simulink library "RoboticsPlayground"  (R2021a)
settings: Solver=FixedStepDiscrete  StartTime=0.0  StopTime=10.0  FixedStep=0.01  RelTol=1e-3
InitFcn:
  | RPInit
undefined symbols (not defined in the file or in its folder): Base, ChassisCOG, Claw2Block1, Claw2Block2, FloorSurface, Frame, PlowSurface, Ref, RobotSurface, Side1, Side2, Wheel2Ground, X, Y, Z
libraries: sm_lib x198, nesl_utility x43, RP_Simulator_Components x23, simulink x2, pid_lib x1
(part 1 of 7)
settings Model: Creator=josea  LastModifiedBy=Sebastian
settings SolverCC: AlgebraicLoopSolver=TrustRegion
settings DataIOCC: ReturnWorkspaceOutputs=off
settings DebuggingCC: SFMachineParentedDataDiag=warning  ArithmeticOperatorsInVariantConditions=warning
settings SFSimCC: SimUseLocalCustomCode=off  CustomCodeUndefinedFunction=UseInterfaceOnly
settings RTWCC: RTWUseLocalCustomCode=off

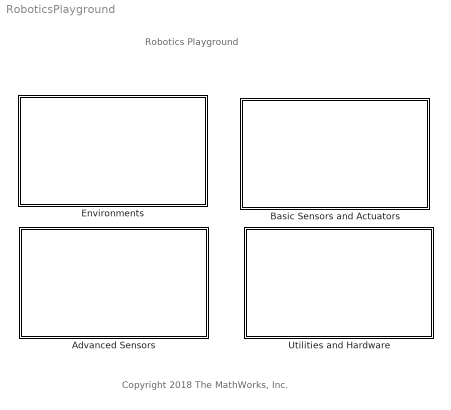
== system RoboticsPlayground ==
  note: Robotics Playground
  note: Copyright 2018 The MathWorks, Inc.
  Advanced Sensors : Subsystem
      mask Display: image('advanced_sensors_lib.PNG')
  Basic Sensors and Actuators : Subsystem
      mask Display: image('sensors_lib.PNG')
  Environments : Subsystem
      mask Display: image('environments_lib.PNG')
  Utilities and Hardware : Subsystem

== system RoboticsPlayground/Advanced Sensors ==
  note: Advanced Sensors
      |
      | Use one of this blocks for each device
  360 Range Sensor : Subsystem  mask(RP 360 Sensor){robotId=1, maxSenRange=2, sensOff=[0 0], sensDegRes=1, sensorTs=0.1}
      mask prompts: robotId "Robot ID"; maxSenRange "Maximum Range (m)"; sensOff "Sensor Position Offset X Y [m]"; sensDegRes "Angular Resolution [deg]"; sensorTs "Sensor sample time [s]"
      mask help:
      | This sensor outputs the ranges measured by a distance sensor at multiple angles of rotation. This sensor can detect walls and obstacles within the simulation environments.
      |
      | The block outputs an array with variable dimensions depending and corresponding to the angular sensor resolution. An angular resolution of 1 degree means the block will output an array of 360 elements each corresponding to the respective ranges at angles from 0 to 359 degrees.
      |
      | NOTE: This block has no visualization in the virtual environment.
      mask init:
      | ID=get_param(gcb,'robotId');
      | 
      | set_param([gcb '/xPose'],'GotoTag',['R' ID 'xPose']);
      | set_param([gcb '/yPose'],'GotoTag',['R' ID 'yPose']);
      | set_param([gcb '/tPose'],'GotoTag',['R' ID 'tPose']);
      mask Help: web('360_sensor.htm')
      mask DialogControl senCont Prompt: Sensor Characteristics
      mask Display:
      | color('white');
      | plot([100,100,100,100]*1,[100,100,100,100]*1);
      | plot([100,100,100,100]*0,[100,100,100,100]*0);
      | image('Lidar.png')
      | color('blue');
      | id=eval(get_param(gcb,'robotId'));
      | text(99, 92, ['Robot ID: ' num2str(id)], 'horizontalAlignment', 'right');
  Object Detector : Subsystem  mask(RP Object Sensor){robotId=1, maxSenRange=2, sensFOV=90, sensOff=[0 0], sensOffDeg=0, sensorTs=0.1}
      mask prompts: robotId "Robot ID"; maxSenRange "Maximum Range (m)"; sensFOV "Sensor Field of View [deg]"; sensOff "Sensor Position Offset X Y [m]"; sensOffDeg "Sensor Orientation Offset [deg]"; sensorTs "Sensor sample time [s]"
      mask help:
      | This block returns information from all the objects that are in the field of vision of the sensor.
      |
      | The output of this block is a variable sized depending on the number of objects that are in sight.
      |
      | This block outputs the [ranges angles labels] of the identified objects. Use the "Pick color" block in the Robotics Playground library to obtain information about a single object.
      |
      | Please refer to the detailed documentation by pressing the "Help" button.
      mask init:
      | ID=get_param(gcb,'robotId');
      | 
      | set_param([gcb '/xPose'],'GotoTag',['R' ID 'xPose']);
      | set_param([gcb '/yPose'],'GotoTag',['R' ID 'yPose']);
      | set_param([gcb '/tPose'],'GotoTag',['R' ID 'tPose']);
      mask Help: web('object_sensor.htm')
      mask DialogControl senCont Prompt: Sensor Characteristics
      mask Display:
      | color('white');
      | plot([100,100,100,100]*1,[100,100,100,100]*1);
      | plot([100,100,100,100]*0,[100,100,100,100]*0);
      | image('ObjectDetector.png','center')
      | color('blue');
      | id=eval(get_param(gcb,'robotId'));
      | text(99, 92, ['Robot ID: ' num2str(id)], 'horizontalAlignment', 'right');
      | color('black')
      | port_label('output', 1', 'Objects');
  Pick Color : Subsystem  mask(RP Pick Color){colorSelection=Red}
      mask prompts: colorSelection "Color"
      mask help: This block receives all the detections from the output of a RP Object Detector and outputs the angle in degrees and distance in meters to the nearest object of the selected color.
      mask init:
      | colorSelection=get_param(gcb,'colorSelection');
      | 
      | if strcmp(colorSelection,'Red')
      |     color=1;
      | elseif strcmp(colorSelection,'Green')
      |     color=2;
      | else
      |     color=3;
      | end
      mask Help: web('pick_color.htm')
      mask TypeOptions colorSelection: Red | Green | Blue
      mask Display:
      | colorSelection=get_param(gcb,'colorSelection');
      | 
      | if strcmp(colorSelection,'Red')
      |     image('RedObjD.png','center')
      | elseif strcmp(colorSelection,'Green')
      |     image('GreenObjD.png','center')
      | else
      |     image('BlueObjD.png','center')
      | end
      | 
      | color('black');
      | port_label('input', 1', 'Objects');
      | port_label('output', 1', 'Angle');
      | port_label('output', 2', 'Distance');

== system RoboticsPlayground/Basic Sensors and Actuators ==
  note: Basic Sensors and Actuators
      |
      | Use one of this blocks for each device
  Compass Sensor : Subsystem  mask(RP Compass Sensor){robotId=1, sensorTs=0.1}
      mask prompts: robotId "Robot ID"; sensorTs "Sensor sample time [s]"
      mask help: This sensor outputs the rotation in degrees as measured from the robot center relative to the world coordinate frame.
      mask init:
      | ID=get_param(gcb,'robotId');
      | 
      | set_param([gcb '/tRate'],'GotoTag',['R' ID 'tAngle']);
      mask Help: web('compass_sensor.htm')
      mask DialogControl senCont Prompt: Sensor Characteristics
      mask Display:
      | color('white');
      | plot([100,100,100,100]*1,[100,100,100,100]*1);
      | plot([100,100,100,100]*0,[100,100,100,100]*0);
      | image('Compass.png','center')
      | color('blue');
      | id=eval(get_param(gcb,'robotId'));
      | text(99, 92, ['Robot ID: ' num2str(id)], 'horizontalAlignment', 'right');
  Contact Switch : Subsystem  mask(RP Contact Switch){robotId=1, trigDist=0.02, sensOff=[0 0], sensOffDeg=0, sensorTs=0.1}
      mask prompts: robotId "Robot ID"; trigDist "Trigger Distance [m]"; sensOff "Sensor Position Offset X Y [m]"; sensOffDeg "Sensor Orientation Offset [deg]"; sensorTs "Sensor sample time [s]"
      mask help:
      | This block outputs 1 if the sensor comes in close proximity to a wall or obstacle. Otherwise it outputs zero. The proximity at which the sensor is triggered can be set through the mask using the "Trigger Distance" field. Default values can also be used.
      |
      | Sensor position and orientation offsets are with respect to the robot center.
      mask init:
      | ID=get_param(gcb,'robotId');
      | 
      | set_param([gcb '/xPose'],'GotoTag',['R' ID 'xPose']);
      | set_param([gcb '/yPose'],'GotoTag',['R' ID 'yPose']);
      | set_param([gcb '/tPose'],'GotoTag',['R' ID 'tPose']);
      mask Help: web('contact_switch.htm')
      mask DialogControl senCont Prompt: Sensor Characteristics
      mask Display:
      | color('white');
      | plot([100,100,100,100]*1,[100,100,100,100]*1);
      | plot([100,100,100,100]*0,[100,100,100,100]*0);
      | image('ContactSwitch.png','center')
      | color('blue');
      | id=eval(get_param(gcb,'robotId'));
      | text(99, 92, ['Robot ID: ' num2str(id)], 'horizontalAlignment', 'right');
  Distance Sensor : Subsystem  mask(RP Distance Sensor){robotId=1, maxSenRange=2, minSenRange=0.02, senRes=0.01, sensOff=[0 0], sensOffDeg=0, sensorTs=0.1}
      mask prompts: robotId "Robot ID"; maxSenRange "Maximum Range (m)"; minSenRange "Minimum Range (m)"; senRes "Resolution (m)"; sensOff "Sensor Position Offset X Y [m]"; sensOffDeg "Sensor Orientation Offset [deg]"; sensorTs "Sensor sample time [s]"
      mask help:
      | This block returns the distance to a nearby object such as walls and obstacles. Several sensor properties can be adjusted from the block mask, but default values can also be used.
      |
      | Sensor position and orientation are with respect to the robot center. Press the help button for more details on block parameters.
      mask init:
      | ID=get_param(gcb,'robotId');
      | 
      | set_param([gcb '/xPose'],'GotoTag',['R' ID 'xPose']);
      | set_param([gcb '/yPose'],'GotoTag',['R' ID 'yPose']);
      | set_param([gcb '/tPose'],'GotoTag',['R' ID 'tPose']);
      mask Help: web('distance_sensor.htm')
      mask DialogControl senCont Prompt: Sensor Characteristics
      mask Display:
      | color('white');
      | plot([100,100,100,100]*1,[100,100,100,100]*1);
      | plot([100,100,100,100]*0,[100,100,100,100]*0);
      | image('ultrasonic_sensor.jpg','center')
      | color('blue');
      | id=eval(get_param(gcb,'robotId'));
      | text(99, 92, ['Robot ID: ' num2str(id)], 'horizontalAlignment', 'right');
  Encoder : Subsystem  mask(RP Motor Encoder){robotId=1, motorChoice=1, rstChoice=No reset, ticks=180, detectDir=off, sensorTs=0.1}
      mask prompts: robotId "Robot ID"; motorChoice "Motor encoder number"; rstChoice "Reset option"; ticks "Ticks per rotation"; detectDir "Detect direction of rotation"; sensorTs "Sensor sample time [s]"
      mask help:
      | This block outputs the rotation in tick counts of an encoder conneted to the respective robot motor. You can set different sensor parameters from the mask or use the default settings.
      |
      | The most common use of motor encoders is to derive the position of an object. Start by converting the tick counts to revolutions of the motor shaft. You can later relate the revolutions of the motor shaft to more valuable robot information such as traveled distance by using robot dimensions like the wheel size.
      mask init:
      | blk=gcb;
      | ID = get_param(blk,'robotId');
      | motor = get_param(blk,'motorChoice');
      | 
      | set_param([blk '/motorw'],'GotoTag',['R' ID 'motor' motor 'w']);
      | 
      | 
      | switch get_param(blk,'rstChoice');
      | 
      |     case 'Reset by external signal'
      |         % Check for ground
      |      if strcmp(get_param([blk '/reset'],'BlockType'),'Ground')
      |             replace_block([blk '/reset'],'Ground','Inport','noprompt');
      |      end
      |     case 'No reset'
      |         % Check for inport
      |      if strcmp(get_param([blk '/reset'],'BlockType'),'Inport')
      |             replace_block([blk '/reset'],'Inport','Ground','noprompt')
      |      end
      | end
      mask Help: web('encoder_sensor.htm')
      mask TypeOptions rstChoice: No reset | Reset by external signal
      mask DialogControl ParameterGroupVar Prompt: Settings
      mask Display:
      | color('white');
      | plot([100,100,100,100]*1,[100,100,100,100]*1);
      | plot([100,100,100,100]*0,[100,100,100,100]*0);
      | image('encoder.jpg','center')
      | color('blue');
      | id=eval(get_param(gcb,'robotId'));
      | text(99, 92, ['Robot ID: ' num2str(id)], 'horizontalAlignment', 'right');
  Gyro Sensor : Subsystem  mask(RP Gyro Sensor){robotId=1, sensor=Body Center, sensorTs=0.1}
      mask prompts: robotId "Robot ID"; sensor "Sensor Position"; sensorTs "Sensor sample time [s]"
      mask help:
      | This sensor outputs the rate of rotation in deg/s as measured from a particular sensing point in a robot. You can select different measurement points from the sensor dropdown in the block mask.
      |
      | NOTE: This block has no visualization in the virtual environment.
      mask init:
      | ID=get_param(gcb,'robotId');
      | 
      | set_param([gcb '/tRate'],'GotoTag',['R' ID 'tRate']);
      mask Help: web('gyro_sensor.htm')
      mask TypeOptions sensor: Body Center
      mask DialogControl senCont Prompt: Sensor Characteristics
      mask Display:
      | color('white');
      | plot([100,100,100,100]*1,[100,100,100,100]*1);
      | plot([100,100,100,100]*0,[100,100,100,100]*0);
      | image('Gyroscope.png','center')
      | color('blue');
      | id=eval(get_param(gcb,'robotId'));
      | text(99, 92, ['Robot ID: ' num2str(id)], 'horizontalAlignment', 'right');
  Robot Motor : Subsystem  mask(RP Robot Motor){robotId=1, motorChoice=1}
      mask prompts: robotId "Robot ID"; motorChoice "Motor number"
      mask help:
      | This blocks sets the speed of the respective robot motor. The input is a number in the range of -127 to 127.
      |
      | Refer to environment blocks for motor mapping of different robots.
      mask init:
      | motorCheck(gcs,gcb);
      | ID = get_param(gcb,'robotId');
      | motor = get_param(gcb,'motorChoice');
      | 
      | set_param([gcb '/Goto'],'GotoTag',['R' ID 'motor' motor 't']);
      mask Help: web('motor.htm')
      mask Display:
      | color('white');
      | plot([100,100,100,100]*1,[100,100,100,100]*1);
      | plot([100,100,100,100]*0,[100,100,100,100]*0);
      | image('GlobeMotor.png','center');
      | color('blue');
      | id=eval(get_param(gcb,'robotId'));
      | text(99, 92, ['Robot ID: ' num2str(id)], 'horizontalAlignment', 'right');

== system RoboticsPlayground/Environments ==
  note: Environments
      |
      | Use only one of this environment blocks per model
  note: Copyright 2020 The MathWorks, Inc.
  Clawbot Environment : Subsystem
      mask Display:
      | image('ClawbotIcon.png')
      | port_label('input',1,'leftWheel')
      | port_label('input',2,'rightWheel')
      | port_label('input',3,'armPose')
      | port_label('input',4,'clawPose')
      | port_label('output',1,'xPose')
      | port_label('output',2,'yPose')
      | port_label('output',3,'theta')
      | port_label('output',4,'objectPose')
  MATLAB Disc Robot : Subsystem  mask(RP MATLAB Environment){arenaLength=5, arenaWidth=8, wheelBase=0.5, wheelRadius=0.1, robotColor=[0.5 0 0], startPose=[-1.4 0]}
      mask prompts: arenaLength "Length [m]"; arenaWidth "Width [m]"; wheelBase "Distance between wheels [m]"; wheelRadius "Wheel radius [m]"; robotColor "Color [R G B]"; startPose "Start Position X Y [m]"
      mask help:
      | This block contains a virtual environment with an interface to MATLAB to interact with robot using the MATLAB command line and scripts. It provides the following functionality through MATLAB commands:
      |
      | - Set motor voltages
      | - Read wheel speeds
      | - Read compass angle with respect to the world
      |
      | Please refer to the MATLAB documentation for MLROBOT.
      |
      | Type the following in the MATLAB command prompt:
      |
      | >> help mlrobot
      | >> edit mlrobot_getting_started
      settings: CopyFcn=|
      | set_param(gcs,'InitFcn','RPInit');
      | set_param(gcs,'Solver','ode23t');
      | set_param(gcs, 'EnablePacing', 'on')
      | set_param(gcs, 'PacingRate', 1)
      mask Help: web('MATLAB_robot.htm')
      mask DialogControl Container6 Prompt: Arena settings
      mask DialogControl Container4 Prompt: Robot settings
      mask Display: image('MLRobot.PNG')
  Object Environment : Subsystem  mask(RP Object Environment){obj1=on, objPose1=[0 0], objColor1=Red, obj2=off, objPose2=[0 1], objColor2=Green, obj3=off, objPose3=[0 -1], objColor3=Blue, obj4=off, objPose4=[-0.61298      2.9263], objColor4=Red, obj5=off, objPose5=[-0.61298      2.9263], objColor5=Red, arenaLength=5, arenaWidth=5, robotId=1, wheelBase=0.5, wheelRadius=0.1, robotColor=[0.5 0 0], startPose=[-1.4 0]}
      mask prompts: obj1 "Enabled"; objPose1 "Initial position X Y [m]"; objColor1 "Color"; obj2 "Enabled"; objPose2 "Initial position X Y [m]"; objColor2 "Color"; obj3 "Enabled"; objPose3 "Initial position X Y [m]"; objColor3 "Color"; obj4 "Enabled"; objPose4 "Initial position X Y [m]"; objColor4 "Color"; obj5 "Enabled"; objPose5 "Initial position X Y [m]"; objColor5 "Color"; arenaLength "Length [m]"; arenaWidth "Width [m]"; robotId "Robot ID"; wheelBase "Distance between wheels [m]"; wheelRadius "Wheel radius [m]"; robotColor "Color [R G B]"; startPose "Initial Position X Y [m]"
      mask help:
      | This block contains a virtual environment for a single robot to interact with walls, and objects. Sensors implemented in the Robotics Playground library can be used to obtain environment information and actuators to interact with the robot behavior.
      |
      | Motor mapping for the robot is as follows:
      |
      | Motor 1 -> Left wheel motor torque
      | Motor 2 -> Right wheel motor torque
      settings: CopyFcn=|
      | set_param(gcs,'InitFcn','RPInit');
      | set_param(gcs,'Solver','ode23t');
      | set_param(gcs, 'EnablePacing', 'on')
      | set_param(gcs, 'PacingRate', 1)
      mask Help: web('object_arena.htm')
      mask Callback obj1: setObjects(gcb)
      mask Callback objPose1: setObjects(gcb)
      mask TypeOptions objColor1: Red | Green | Blue
      mask Callback objColor1: setObjects(gcb)
      mask Callback obj2: setObjects(gcb)
      mask Callback objPose2: setObjects(gcb)
      mask TypeOptions objColor2: Red | Green | Blue
      mask Callback objColor2: setObjects(gcb)
      mask Callback obj3: setObjects(gcb)
      mask Callback objPose3: setObjects(gcb)
      mask TypeOptions objColor3: Red | Green | Blue
      mask Callback objColor3: setObjects(gcb)
      mask Callback obj4: setObjects(gcb)
      mask Callback objPose4: setObjects(gcb)
      mask TypeOptions objColor4: Red | Green | Blue
      mask Callback objColor4: setObjects(gcb)
      mask Callback obj5: setObjects(gcb)
      mask Callback objPose5: setObjects(gcb)
      mask TypeOptions objColor5: Red | Green | Blue
      mask Callback objColor5: setObjects(gcb)
      mask DialogControl objT Prompt: Object settings
      mask DialogControl objc1 Prompt: Object 1
      mask DialogControl objc2 Prompt: Object 2
      mask DialogControl objc3 Prompt: Object 3
      mask DialogControl objc4 Prompt: Object 4
      mask DialogControl objc5 Prompt: Object 5
      mask DialogControl Container6 Prompt: Arena settings
      mask DialogControl Container4 Prompt: Robot settings
      mask Display:
      | color('white');
      | plot([100,100,100,100]*1,[100,100,100,100]*1);
      | plot([100,100,100,100]*0,[100,100,100,100]*0);
      | image('ObjectEnv.PNG')
      | color('blue');
      | id=eval(get_param(gcb,'robotId'));
      | text(99, 92, ['Robot ID: ' num2str(id)], 'horizontalAlignment', 'right');
  Obstacle Environment : Subsystem  mask(RP Obstacle Environment){obstacles=[9.31 7.93 9.17 1.22;4.5 13.07 1.22 3.54;6.6 15.39 2.71 1.05;7.6 12.68 1.44 1.71;17.49 15.22 3.65 0.94;22.4 12.62 1.55 3.15;18.48 12.9 1.99 1.49;18.87 3.07 1.44 5.64;12.29 1.91 5.36 1.55;7.87 3.45 4.25 0.5;6.05 3.56 0.94 9.23;9.97 12.07 1.55 3.54;12.62 11.63 6.57 0.77;26.49 14.72 1.77 2.93;27.87 5.11 0.66 6.35;26.66 0.69 2.1 1.88;1.74 0.75 1.44 2.21;1.13 17.21 1.88 1.66;1.69 9.53 1.27 2.65;13.84 17.76 1.44 1.1;21.74 17.71 2.65 1.16], arenaLength=30, arenaWidth=20, robotId=1, wheelBase=0.5, wheelRadius=0.1, robotColor=[0.5 0 0], startPose=[-1.4 0]}
      mask prompts: obstacles "Obstacles matrix[nx4] with rectangles with the form [x,y,length,width]"; arenaLength "Length [m]"; arenaWidth "Width [m]"; robotId "Robot ID"; wheelBase "Distance between wheels [m]"; wheelRadius "Wheel radius [m]"; robotColor "Color [R G B]"; startPose "Initial Position X Y [m]"
      mask help:
      | This block contains a virtual environment for a single robot to interact with walls, obstacles and objects. Sensors implemented in the Robotics Playground library can be used to obtain environment information and actuators to interact with the robot behavior.
      |
      | Motor mapping for the robot is as follows:
      |
      | Motor 1 -> Left wheel motor torque
      | Motor 2 -> Right wheel motor torque
      settings: CopyFcn=|
      | set_param(gcs,'InitFcn','RPInit');
      | set_param(gcs,'Solver','ode23t');
      | set_param(gcs, 'EnablePacing', 'on')
      | set_param(gcs, 'PacingRate', 1)
      mask Help: web('obstacle_arena.htm')
      mask DialogControl obsT Prompt: Obstacle settings
      mask DialogControl Container19 Prompt: Set Obstacles Interactively
      mask DialogControl Control2 Prompt: Set Obstacles
      mask DialogControl Control2 Callback: setObstaclesUI(gcb)
      mask DialogControl Container6 Prompt: Arena settings
      mask DialogControl Container4 Prompt: Robot settings
      mask Display:
      | color('white');
      | plot([100,100,100,100]*1,[100,100,100,100]*1);
      | plot([100,100,100,100]*0,[100,100,100,100]*0);
      | image('ObstacleEnv.PNG')
      | color('blue');
      | id=eval(get_param(gcb,'robotId'));
      | text(99, 92, ['Robot ID: ' num2str(id)], 'horizontalAlignment', 'right');
  Sumo Game : Subsystem  mask(RP Sumo Game){arenaLength=5, arenaWidth=5, circleRadius=1.8, difficulty=Medium, robot1Id=1, startPose1=[-0.4 0], wheelBase1=0.5, wheelRadius1=0.1, color1=[0 0 0.5], robot2Id=2, startPose2=[0.4 0], wheelBase2=0.5, wheelRadius2=0.1, color2=[0.5 0 0]}
      mask prompts: arenaLength "Length [m]"; arenaWidth "Width [m]"; circleRadius "Sumo circle radius [m]"; robot1Id "Robot ID"; startPose1 "Initial position X Y [m]"; wheelBase1 "Distance between wheels [m]"; wheelRadius1 "Wheel radius [m]"; color1 "Color [R G B]"; robot2Id "Robot ID"; startPose2 "Initial position X Y [m]"; wheelBase2 "Distance between wheels [m]"; wheelRadius2 "Wheel radius [m]"; color2 "Color"
      mask help:
      | This is a fully imlpemented simulation environment for a robot sumo game. The goal of the game is for one of the robots to push the competitor outside of the area bounded by the circle. Provide input torques to the motors through motor blocks in order to control the robot behavior.
      |
      | Motor mappings for both the robots are as follows:
      |
      | Motor 1 -> Left wheel force
      | Motor 2 -> Right wheel force
      mask init:
      | diff=get_param(gcb,'difficulty');
      | if strcmp(diff,'Medium')
      |     maxTorque=6;
      | elseif strcmp(diff,'Hard')
      |     maxTorque=9;
      | else
      |     maxTorque=3;
      | end
      | 
      | % Check robot ID's are different
      | blk=gcb;
      | id1=get_param(blk,'robot1Id');
      | id2=get_param(blk,'robot2Id');
      | 
      | if id1 == id2
      |     error('Please make sure robot ID''s are different')
      | end
      settings: CopyFcn=|
      | set_param(gcs,'InitFcn','RPInit');
      | set_param(gcs,'Solver','ode23t');
      | set_param(gcs, 'EnablePacing', 'on')
      | set_param(gcs, 'PacingRate', 1)
      mask Help: web('sumo_game.htm')
      mask TypeOptions difficulty: Easy | Medium | Hard
      mask DialogControl Container5 Prompt: Game settings
      mask DialogControl Container8 Prompt: Robot 1 settings
      mask DialogControl Container9 Prompt: Robot 2 settings
      mask Display:
      | color('white');
      | plot([100,100,100,100]*1,[100,100,100,100]*1);
      | plot([100,100,100,100]*0,[100,100,100,100]*0);
      | image('SumoGame.PNG')
      | color('blue');
      | id=eval(get_param(gcb,'robot1Id'));
      | text(99, 92, ['Robot 1 ID: ' num2str(id)], 'horizontalAlignment', 'right');
      | id=eval(get_param(gcb,'robot2Id'));
      | text(99, 82, ['Robot 2 ID: ' num2str(id)], 'horizontalAlignment', 'right');

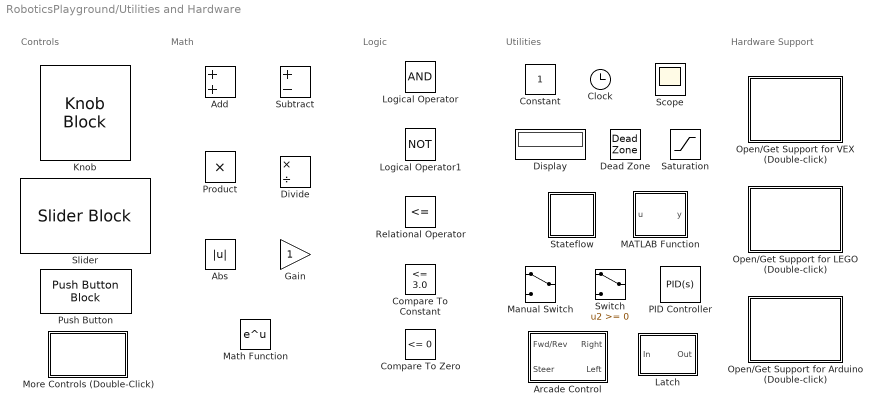
== system RoboticsPlayground/Utilities and Hardware ==
  note: Controls
  note: Hardware Support
  note: Math
  note: Logic
  note: Utilities
  Abs : Abs
  Add : Sum
  Arcade Control : Subsystem
      mask Display:
      | image('arcadeModule.png')
      | port_label('input',1,'Fwd/Rev')
      | port_label('input',2,'Steer')
      | port_label('output',2,'LeftMotor')
      | port_label('output',1,'RightMotor')
  Clock : Clock
  Compare To Constant : simulink/Logic and Bit Operations/Compare To Constant  relop=<=  const=3.0  OutDataTypeStr=boolean
  Compare To Zero : simulink/Logic and Bit Operations/Compare To Zero  relop=<=  OutDataTypeStr=boolean
  Constant : Constant
  Dead Zone : DeadZone  SaturateOnIntegerOverflow=on
  Display : Display
  Divide : Product  Inputs=*/
  Gain : Gain
  Knob : KnobBlock
  Latch : Subsystem
      mask Display:
      | image('latchGraph.png')
      | port_label('input',1,'In')
      | port_label('output',1,'Out')
  Logical Operator : Logic  AllPortsSameDT=off  OutDataTypeStr=boolean
  Logical Operator1 : Logic  Operator=NOT  AllPortsSameDT=off  OutDataTypeStr=boolean
  MATLAB Function : MATLAB Function  TreatAsAtomicUnit=on
  Manual Switch : ManualSwitch
  Math Function : Math  SignedPower=on  SaturateOnIntegerOverflow=on
  More Controls (Double-Click) : Subsystem
      settings: OpenFcn=open_system('Simulink/Dashboard')
      mask Display: disp(get_param(gcb,'name'))
  Open/Get Support for Arduino (Double-click) : Subsystem
      settings: OpenFcn=|
      | try
      |    open_system('arduinolib');
      | catch
      |     message=sprintf(['Please get the Simulink support package for Arduino from the following url:\n\n' 'https://www.mathworks.com/hardware-support/arduino-simulink.html' '\n\nPress OK to open the URL']);
      |     uiwait(msgbox(message,'Get Simulink Arduino support package'));
      |     web('https://www.mathworks.com/hardware-support/arduino-simulink.html','-browser');
      | end
      mask Display: disp(get_param(gcb,'name'))
  Open/Get Support for LEGO (Double-click) : Subsystem
      settings: OpenFcn=|
      | try
      |    open_system('legoev3lib') ;
      | catch
      |     message=sprintf(['Please get the Simulink support package for LEGO EV3 hardware from the following url:\n\n' 'https://www.mathworks.com/hardware-support/lego-mindstorms-ev3-simulink.html' '\n\nPress OK to open the URL']);
      |     uiwait(msgbox(message,'Get Simulink LEGO support package'));
      |     web('https://www.mathworks.com/hardware-support/lego-mindstorms-ev3-simulink.html','-browser');
      | end
      mask Display: disp(get_param(gcb,'name'))
  Open/Get Support for VEX (Double-click) : Subsystem
      settings: OpenFcn=|
      | try
      |    open_system('vexarmcortexlib');
      | catch
      |     message=sprintf(['Please get the Simulink support package for VEX hardware from the following url:\n\n' 'https://www.mathworks.com/hardware-support/vex-arm-cortex.html' '\n\nPress OK to open the URL']);
      |     uiwait(msgbox(message,'Get Simulink VEX support package'));
      |     web('https://www.mathworks.com/hardware-support/vex-arm-cortex.html','-browser');
      | end
      mask Display: disp(get_param(gcb,'name'))
  PID Controller : pid_lib/PID Controller  Controller=PID  Form=Parallel  TimeDomain=Continuous-time  UseExternalTs=off  SampleTime=-1  IntegratorMethod=Forward Euler  FilterMethod=Forward Euler  ControllerParametersSource=internal  P=1  I=1  D=0  UseFilter=on  N=100  TunerSelectOption=Transfer Function Based (PID Tuner App)  InitialConditionSource=internal  InitialConditionForIntegrator=0  InitialConditionForFilter=0  DifferentiatorICPrevScaledInput=0  ExternalReset=none  TrackingMode=off  Kt=1  LimitOutput=off  SatLimitsSource=internal  UpperSaturationLimit=inf  LowerSaturationLimit=-inf  LinearizeAsGain=on  AntiWindupMode=none  Kb=1  POutMin=[]  POutMax=[]  IOutMin=[]  IOutMax=[]  DOutMin=[]  DOutMax=[]  NOutMin=[]  NOutMax=[]  SumOutMin=[]  SumOutMax=[]  SaturationOutMin=[]  SaturationOutMax=[]  PParamMin=[]  PParamMax=[]  IParamMin=[]  IParamMax=[]  DParamMin=[]  DParamMax=[]  NParamMin=[]  NParamMax=[]  KbParamMin=[]  KbParamMax=[]  KtParamMin=[]  KtParamMax=[]  KbOutMin=[]  KbOutMax=[]  KtOutMin=[]  KtOutMax=[]  IntegratorOutMin=[]  IntegratorOutMax=[]  FilterOutMin=[]  FilterOutMax=[]  SumI1OutMin=[]  SumI1OutMax=[]  SumI2OutMin=[]  SumI2OutMax=[]  SumI3OutMin=[]  SumI3OutMax=[]  SumI4OutMin=[]  SumI4OutMax=[]  SumDOutMin=[]  SumDOutMax=[]  DifferentiatorOutMin=[]  DifferentiatorOutMax=[]  FilterDiffOutCoefMin=[]  FilterDiffOutCoefMax=[]  ReciprocalOutMin=[]  ReciprocalOutMax=[]  SumDenOutMin=[]  SumDenOutMax=[]  SumNumOutMin=[]  SumNumOutMax=[]  DivideOutMin=[]  DivideOutMax=[]  UdiffTsProdOutMin=[]  UdiffTsProdOutMax=[]  NTsProdOutMin=[]  NTsProdOutMax=[]  UintegralTsProdOutMin=[]  UintegralTsProdOutMax=[]  UngainTsProdOutMin=[]  UngainTsProdOutMax=[]  IntegratorContinuousStateAttributes=''  IntegratorStateMustResolveToSignalObject=off  IntegratorRTWStateStorageClass=Auto  FilterContinuousStateAttributes=''  FilterStateMustResolveToSignalObject=off  FilterRTWStateStorageClass=Auto  ParallelPVariant=InternalParameters  IdealPVariant=Disabled  IVariant=InternalParameters  DVariant=InternalParameters  IntegratorVariant=Continuous  SatVariant=Disabled  AWVariant=Passthrough  PCopyVariant=Disabled  TRVariant=Disabled  FdbkBlocksVariant=Forward  IdealPFdbkVariant=Disabled  SatFdbkVariant=Disabled  DerivativeFilterVariant=ContFilter  NVariant=InternalParameters  NCopyVariant=Disabled  FilterICVariant=InternalICsFilter  IntegratorICVariant=InternalICs  ExternalResetVariant=Disabled  TRSumVariant=Passthrough  SumFdbkVariant=Disabled  SumVariant=Sum_PID  TsampFilterVariant=InternalTs  TsampNgainVariant=Passthrough  TsampIntegralVariant=Passthrough  ExternalSaturationOutDataTypeStr=Inherit: Same as second input
  Product : Product  RndMeth=Zero
  Push Button : PushButtonBlock  LabelPosition=Top
  Relational Operator : RelationalOperator  Operator=<=  OutDataTypeStr=boolean  RndMeth=Nearest
  Saturation : Saturate
  Scope : Scope
  Slider : SliderBlock
  Stateflow : Stateflow chart  TreatAsAtomicUnit=on
  Subtract : Sum  Inputs=+-
  Switch : Switch

== system RoboticsPlayground/Advanced Sensors/360 Range Sensor ==
  MATLAB System : MATLABSystem  System=LidarSensorRP  mapName=occGrid  sensorOffset=sensOff  scanAngles=[ 0:sensDegRes*pi/180:2*pi-(sensDegRes*pi/180)]  maxRange=maxSenRange
      mask Type: LidarSensorRP
      mask Display:
      | disp(['Lidar' char(10) 'Sensor']);
      | port_label('input',1,'pose');
      | port_label('output',1,'ranges');
  Mux : Mux  Inputs=3
  Rate Transition1 : RateTransition  OutPortSampleTime=sensorTs
  Distance : Outport  VectorParamsAs1DForOutWhenUnconnected=off
  wires:
  Mux/1 -> Rate Transition1/1
  [R1tPose] -> Mux/3
  [R1yPose] -> Mux/2
  [R1xPose] -> Mux/1
  MATLAB System/1 -> Distance/1
  Rate Transition1/1 -> MATLAB System/1

== system RoboticsPlayground/Advanced Sensors/Object Detector ==
  Mux : Mux  Inputs=3
  Object Detector Src : MATLABSystem  System=ObjectDetectorRP  mapName=occGrid  sensorOffset=sensOff  sensorAngle=sensOffDeg*pi/180  fieldOfView=sensFOV*pi/180  maxRange=maxSenRange  maxDetections=5
      mask Type: ObjectDetectorRP
      mask Display:
      | disp(['Object' char(10) 'Detector']);
      | port_label('input',1,'pose');
      | port_label('input',2,'objects');
      | port_label('output',1,'detections');
  Rate Transition : RateTransition  OutPortSampleTime=sensorTs
  Subsystem : Subsystem
  Distance : Outport  VectorParamsAs1DForOutWhenUnconnected=off
  wires:
  Mux/1 -> Rate Transition/1
  [R1tPose] -> Mux/3
  [R1yPose] -> Mux/2
  [R1xPose] -> Mux/1
  Object Detector Src/1 -> Distance/1
  Rate Transition/1 -> Object Detector Src/1
  Subsystem/1(Objects) -> Object Detector Src/2

== system RoboticsPlayground/Advanced Sensors/Pick Color ==
  Objects : Inport
  MATLAB Function : MATLAB Function  TreatAsAtomicUnit=on
  rad2deg : Gain  Gain=180/pi
  Angle : Outport  VectorParamsAs1DForOutWhenUnconnected=off
  Distance : Outport  Port=2  VectorParamsAs1DForOutWhenUnconnected=off
  wires:
  Objects/1 -> MATLAB Function/1(objectsDetected)
  MATLAB Function/1(angle) -> rad2deg/1
  MATLAB Function/2(range) -> Distance/1
  rad2deg/1 -> Angle/1

== system RoboticsPlayground/Basic Sensors and Actuators/Compass Sensor ==
  Rate Transition : RateTransition  OutPortSampleTime=sensorTs
  Distance : Outport  VectorParamsAs1DForOutWhenUnconnected=off
  wires:
  Rate Transition/1 -> Distance/1
  [R1tAngle] -> Rate Transition/1

== system RoboticsPlayground/Basic Sensors and Actuators/Contact Switch ==
  Constant : Constant  Value=trigDist
  MATLAB System : MATLABSystem  System=LidarSensorRP  mapName=occGrid  sensorOffset=sensOff  scanAngles=sensOffDeg*pi/180  maxRange=trigDist+1
      mask Type: LidarSensorRP
      mask Display:
      | disp(['Lidar' char(10) 'Sensor']);
      | port_label('input',1,'pose');
      | port_label('output',1,'ranges');
  Mux : Mux  Inputs=3
  Rate Transition1 : RateTransition  OutPortSampleTime=sensorTs
  Relational Operator : RelationalOperator  Operator=<  OutDataTypeStr=boolean  RndMeth=Nearest
  Distance : Outport  VectorParamsAs1DForOutWhenUnconnected=off
  wires:
  Mux/1 -> Rate Transition1/1
  [R1tPose] -> Mux/3
  [R1yPose] -> Mux/2
  [R1xPose] -> Mux/1
  MATLAB System/1 -> Relational Operator/1
  Constant/1 -> Relational Operator/2
  Relational Operator/1 -> Distance/1
  Rate Transition1/1 -> MATLAB System/1

== system RoboticsPlayground/Basic Sensors and Actuators/Distance Sensor ==
  MATLAB System : MATLABSystem  System=LidarSensorRP  mapName=occGrid  sensorOffset=sensOff  scanAngles=sensOffDeg*pi/180  maxRange=maxSenRange
      mask Type: LidarSensorRP
      mask Display:
      | disp(['Lidar' char(10) 'Sensor']);
      | port_label('input',1,'pose');
      | port_label('output',1,'ranges');
  Mux : Mux  Inputs=3
  Quantizer : Quantizer  QuantizationInterval=senRes
  Rate Transition1 : RateTransition  OutPortSampleTime=sensorTs
  Saturation : Saturate  UpperLimit=maxSenRange  LowerLimit=minSenRange
  Distance : Outport  VectorParamsAs1DForOutWhenUnconnected=off
  wires:
  [R1xPose] -> Mux/1
  [R1yPose] -> Mux/2
  [R1tPose] -> Mux/3
  Mux/1 -> Rate Transition1/1
  MATLAB System/1 -> Quantizer/1
  Quantizer/1 -> Saturation/1
  Saturation/1 -> Distance/1
  Rate Transition1/1 -> MATLAB System/1

== system RoboticsPlayground/Basic Sensors and Actuators/Encoder ==
  Abs : Abs
  Constant : Constant  Value=detectDir
  Gain2 : Gain  Gain=180/pi
  Gain3 : Gain  Gain=ticks/360
  Integrator : Integrator  ExternalReset=rising
  Rate Transition : RateTransition  OutPortSampleTime=sensorTs
  Rounding Function : Rounding  Operator=ceil
  Switch : Switch  Criteria=u2 ~= 0
  reset : Ground
  Out1 : Outport  VectorParamsAs1DForOutWhenUnconnected=off
  wires:
  Abs/1 -> Switch/3
  Constant/1 -> Switch/2
  [R1motor1w] -> Switch/1, Abs/1
  Switch/1 -> Gain2/1
  reset/1 -> Integrator/2
  Integrator/1 -> Gain3/1
  Gain2/1 -> Integrator/1
  Gain3/1 -> Rounding Function/1
  Rounding Function/1 -> Rate Transition/1
  Rate Transition/1 -> Out1/1

== system RoboticsPlayground/Basic Sensors and Actuators/Gyro Sensor ==
  Rate Transition : RateTransition  OutPortSampleTime=sensorTs
  Distance : Outport  VectorParamsAs1DForOutWhenUnconnected=off
  wires:
  [R1tRate] -> Rate Transition/1
  Rate Transition/1 -> Distance/1

== system RoboticsPlayground/Basic Sensors and Actuators/Robot Motor ==
  In1 : Inport
  tag scope: R1motor1t=global
  wires:
  In1/1 -> [R1motor1t]

== system RoboticsPlayground/Environments/Clawbot Environment ==
  note: See examples using this environment:
      | - Clawbot Teleoperation
      | - Clawbot Autonomous
      | - Clawbot Perception
  LeftWheel : Inport
  RightWheel : Inport  Port=2
  armPose : Inport  Port=3
  clawPose : Inport  Port=4
  ClawBot : Subsystem
      mask Display: image('Clawbot Simscape.PNG'); % Use "Edit Image" on toolstrip to change.
  Environment : Subsystem  mask{x_block1=10, y_block1=40, x_goal1=15, y_goal1=70, x_block2=-20, y_block2=110, x_goal2=5, y_goal2=150, target1_radius=4, target1_height=12, target2_radius=3, target2_height=10}
      mask prompts: x_block1 "Block 1 X position"; y_block1 "Block 1 Y position"; x_goal1 "Target 1 X position"; y_goal1 "Target1 Y position"; x_block2 "Block 2 X position"; y_block2 "Block 2 Y position"; x_goal2 "Target 2 X position"; y_goal2 "Target 2 Y position"; target1_radius "Target 1 radius"; target1_height "Target 1 height"; target2_radius "Target 2 radius"; target2_height "Target 2 height"
      mask init:
      | %target = [x_block1 y_block1; x_goal1 y_goal1;x_block2 y_block2;x_goal2 y_goal2];
      | %length_arm = 11.854;
      mask Display: image('Simscape Environment.PNG'); % Use "Edit Image" on toolstrip to change.
  xPose : Outport
  yPose : Outport  Port=2
  theta : Outport  Port=3
  Target Coordinates : Outport  Port=4
  wires:
  ClawBot/1(xPose) -> xPose/1
  ClawBot/2(yPose) -> yPose/1
  RightWheel/1 -> ClawBot/2(RightWheel)
  Environment/1(Targets) -> Target Coordinates/1
  ClawBot/3(theta) -> theta/1
  LeftWheel/1 -> ClawBot/1(LeftWheel)
  clawPose/1 -> ClawBot/4(clawPose)
  armPose/1 -> ClawBot/3(armPose)
  connections:
  ClawBot/LConn1 -- Environment/LConn1

== system RoboticsPlayground/Environments/MATLAB Disc Robot ==
  Obstacle Arena : RP_Simulator_Components/Obstacle Arena  length=arenaLength  width=arenaWidth  robotRadius=wheelBase/2
  Robot : Subsystem  mask(RP Contact Tank Robot){robotId=1, wheelRadius=wheelRadius, wheelBase=wheelBase, wheelThickness=0.025, chassisThickness=0.05, startPose=startPose, choice=off, sensorTs=0.05, wheelMass=0.2, chassisMass=0.5, maxWheelTorque=1, floorSize=[arenaLength arenaWidth], wheelColor=[0.25 0.25 0.25], chassisColor=robotColor}
      mask prompts: robotId "Robot ID"; wheelRadius "Wheel Radius [m]"; wheelBase "Wheelbase [m]"; wheelThickness "Wheel Thickness [m]"; chassisThickness "Chassis Thickness [m]"; startPose "Start Position [m]"; choice "Reverse Start Position"; sensorTs "Sensor sample time [s]"; wheelMass "Wheel Mass [kg]"; chassisMass "Chassis Mass [kg]"; maxWheelTorque "Maximum wheel torque [N*m]"; floorSize "Floor Dimensions [m]"; wheelColor "Wheel Color"; chassisColor "Chassis Color"
      mask help:
      | This robot implements contact between the robot wheels and the floor of an arena. The stck-slip friction implemented using contact force libraries makes the robot behavior more realistic. The inputs to the robot are now motor torque, which is set using the Robotics Playground Motor blocks. The motor mappings are as follows:
      |
      | Motor 1 -> Left wheel motor torque
      | Motor 2 -> Right wheel motor torque
      mask DialogControl KinContainer Prompt: Kinematics
      mask DialogControl DynamicsContainer Prompt: Dynamics
      mask DialogControl AppearanceContainer Prompt: Appearance
      mask Display:
      | image('discRobot.PNG')
      | port_label('Rconn',1,'RP-Bus')
  connections:
  Robot/RConn1 -- Obstacle Arena/LConn1

== system RoboticsPlayground/Environments/Object Environment ==
  Object Arena : RP_Simulator_Components/Object Arena  length=arenaLength  width=arenaWidth  robotRadius=wheelBase/2
  Objects : Subsystem
  Plow Tank Robot : Subsystem  AncestorBlock=RP_Simulator_Components/Plow Tank Robot  mask(RP Contact Tank Robot){robotId=robotId, wheelRadius=wheelRadius, wheelBase=wheelBase, wheelThickness=0.025, chassisThickness=0.05, startPose=startPose, choice=off, sensorTs=0.05, wheelMass=0.2, chassisMass=0.5, maxWheelTorque=1, floorSize=[arenaLength arenaWidth], wheelColor=[0.25 0.25 0.25], chassisColor=robotColor}
      mask prompts: robotId "Robot ID"; wheelRadius "Wheel Radius [m]"; wheelBase "Wheelbase [m]"; wheelThickness "Wheel Thickness [m]"; chassisThickness "Chassis Thickness [m]"; startPose "Start Position [m]"; choice "Reverse Start Position"; sensorTs "Sensor sample time [s]"; wheelMass "Wheel Mass [kg]"; chassisMass "Chassis Mass [kg]"; maxWheelTorque "Maximum wheel torque [N*m]"; floorSize "Floor Dimensions [m]"; wheelColor "Wheel Color"; chassisColor "Chassis Color"
      mask help:
      | This robot implements contact between the robot wheels and the floor of an arena. The stck-slip friction implemented using contact force libraries makes the robot behavior more realistic. The inputs to the robot are now motor torque, which is set using the Robotics Playground Motor blocks. The motor mappings are as follows:
      |
      | Motor 1 -> Left wheel motor torque
      | Motor 2 -> Right wheel motor torque
      mask init:
      | ID=num2str(eval(get_param(gcb,'robotId')));
      | block=gcb;
      | 
      | set_param([block '/motor1t'],'GotoTag',['R' ID 'motor1t']);
      | set_param([block '/motor2t'],'GotoTag',['R' ID 'motor2t']);
      | set_param([block '/motor1q'],'GotoTag',['R' ID 'motor1q']);
      | set_param([block '/motor1w'],'GotoTag',['R' ID 'motor1w']);
      | set_param([block '/motor2q'],'GotoTag',['R' ID 'motor2q']);
      | set_param([block '/motor2w'],'GotoTag',['R' ID 'motor2w']);
      | set_param([block '/xPose'],'GotoTag',['R' ID 'xPose']);
      | set_param([block '/yPose'],'GotoTag',['R' ID 'yPose']);
      | set_param([block '/tPose'],'GotoTag',['R' ID 'tPose']);
      | set_param([block '/tRate'],'GotoTag',['R' ID 'tRate']);
      | set_param([block '/tAngle'],'GotoTag',['R' ID 'tAngle']);
      | 
      | % Add sensor visuals
      | 
      | addSensors(block,eval(ID));
      mask DialogControl KinContainer Prompt: Kinematics
      mask DialogControl DynamicsContainer Prompt: Dynamics
      mask DialogControl AppearanceContainer Prompt: Appearance
      mask Display:
      | image('plowRobot.PNG')
      | port_label('Rconn',1,'RP-Bus')
  connections:
  Objects/LConn1 -- Object Arena/LConn1 -- Plow Tank Robot/RConn1

== system RoboticsPlayground/Environments/Obstacle Environment ==
  Obstacle Arena : RP_Simulator_Components/Obstacle Arena  length=arenaLength  width=arenaWidth  robotRadius=wheelBase/2
      link override Floor/Floor: BrickDimensions=[length width 0.01]
      link override Floor/Grid: grid_origin="[-length  -width 0]"  grid_size=[ length width]
      link override Walls/Rigid Transform: TranslationCartesianOffset=[0 width/2 0]
      link override Walls/Rigid Transform1: TranslationCartesianOffset=[0 -width/2 0]
      link override Walls/Rigid Transform2: TranslationCartesianOffset=[length/2 0 0]
      link override Walls/Rigid Transform3: TranslationCartesianOffset=[-length/2 0 0]
      link override Walls/Wall 1: BrickDimensions=[length 0.04 height]
      link override Walls/Wall 2: BrickDimensions=[length 0.04 height]
      link override Walls/Wall 3: BrickDimensions=[width 0.04 height]
      link override Walls/Wall 4: BrickDimensions=[width 0.04 height]
  Obstacles : Subsystem
  Robot : Subsystem  AncestorBlock=RP_Simulator_Components/Contact Tank Robot  mask(RP Contact Tank Robot){robotId=robotId, wheelRadius=wheelRadius, wheelBase=wheelBase, wheelThickness=0.025, chassisThickness=0.05, startPose=startPose, choice=off, sensorTs=0.05, wheelMass=0.2, chassisMass=0.5, maxWheelTorque=4, floorSize=[arenaLength arenaWidth], wheelColor=[0.25 0.25 0.25], chassisColor=robotColor}
      mask prompts: robotId "Robot ID"; wheelRadius "Wheel Radius [m]"; wheelBase "Wheelbase [m]"; wheelThickness "Wheel Thickness [m]"; chassisThickness "Chassis Thickness [m]"; startPose "Start Position [m]"; choice "Reverse Start Position"; sensorTs "Sensor sample time [s]"; wheelMass "Wheel Mass [kg]"; chassisMass "Chassis Mass [kg]"; maxWheelTorque "Maximum wheel torque [N*m]"; floorSize "Floor Dimensions [m]"; wheelColor "Wheel Color"; chassisColor "Chassis Color"
      mask help:
      | This robot implements contact between the robot wheels and the floor of an arena. The stck-slip friction implemented using contact force libraries makes the robot behavior more realistic. The inputs to the robot are now motor torque, which is set using the Robotics Playground Motor blocks. The motor mappings are as follows:
      |
      | Motor 1 -> Left wheel motor torque
      | Motor 2 -> Right wheel motor torque
      mask init:
      | block=gcb;
      | ID=num2str(eval(get_param(block,'robotId')));
      | 
      | set_param([block '/motor1t'],'GotoTag',['R' ID 'motor1t']);
      | set_param([block '/motor2t'],'GotoTag',['R' ID 'motor2t']);
      | set_param([block '/motor1q'],'GotoTag',['R' ID 'motor1q']);
      | set_param([block '/motor1w'],'GotoTag',['R' ID 'motor1w']);
      | set_param([block '/motor2q'],'GotoTag',['R' ID 'motor2q']);
      | set_param([block '/motor2w'],'GotoTag',['R' ID 'motor2w']);
      | set_param([block '/xPose'],'GotoTag',['R' ID 'xPose']);
      | set_param([block '/yPose'],'GotoTag',['R' ID 'yPose']);
      | set_param([block '/tPose'],'GotoTag',['R' ID 'tPose']);
      | set_param([block '/tRate'],'GotoTag',['R' ID 'tRate']);
      | set_param([block '/tAngle'],'GotoTag',['R' ID 'tAngle']);
      | 
      | % Add sensor visuals
      | 
      | addSensors(block,eval(ID));
      mask DialogControl KinContainer Prompt: Kinematics
      mask DialogControl DynamicsContainer Prompt: Dynamics
      mask DialogControl AppearanceContainer Prompt: Appearance
      mask Display:
      | image('discRobot.PNG')
      | port_label('Rconn',1,'RP-Bus')
  connections:
  Obstacles/LConn1 -- Robot/RConn1 -- Obstacle Arena/LConn1

== system RoboticsPlayground/Environments/Sumo Game ==
  Arena : RP_Simulator_Components/Sumo Arena  length=arenaLength  width=arenaWidth  circleRadius=circleRadius  robotRadius1=wheelBase1/2  robotRadius2=wheelBase2/2
  Robot 1 : RP_Simulator_Components/Simple Tank Robot  robotId=1  wheelRadius=wheelRadius1  wheelBase=wheelBase1  wheelThickness=0.025  chassisThickness=0.05  startPose=startPose1  choice=off  timeConstant=0.05  wheelMass=0.1  chassisMass=1  maxWheelTorque=maxTorque  wheelColor=[0.25 0.25 0.25]  chassisColor=color1
  Robot 2 : RP_Simulator_Components/Simple Tank Robot  robotId=2  wheelRadius=wheelRadius2  wheelBase=wheelBase2  wheelThickness=0.025  chassisThickness=0.05  startPose=startPose2  choice=on  timeConstant=0.05  wheelMass=0.1  chassisMass=1  maxWheelTorque=maxTorque  wheelColor=[0.25 0.25 0.25]  chassisColor=color2
  connections:
  Robot 1/RConn1 -- Arena/LConn1
  Robot 2/RConn1 -- Arena/LConn2

== system RoboticsPlayground/Utilities and Hardware/Arcade Control ==
  note: Provide arcade style control to a tank robot.
      |
      | This block can be used for tank robot control with a single stick, where each axis of the joystick is passed to a different input. One joystick channel controls Forward/Reverse speed and another controls Left/Right Steer differential to provide rotation.
      |
      | The input values are expected to be between -127 and 127 (often they are the outputs of Gamepad Joystick or Gamepad Accelerometer blocks). The output values also range from -127 to 127 (often they are connected to DC Motor blocks).
  Fwd/Rev : Inport
  Steer : Inport  Port=2
  Add : Sum
  Add1 : Sum  Inputs=+-
  Saturation : Saturate  UpperLimit=127  LowerLimit=-127
  Saturation1 : Saturate  UpperLimit=127  LowerLimit=-127
  Right : Outport  VectorParamsAs1DForOutWhenUnconnected=off
  Left : Outport  Port=2  VectorParamsAs1DForOutWhenUnconnected=off
  wires:
  Add1/1 -> Saturation1/1
  Add/1 -> Saturation/1
  Steer/1 -> Add/2, Add1/2
  Fwd/Rev/1 -> Add/1, Add1/1
  Saturation1/1 -> Right/1
  Saturation/1 -> Left/1

== system RoboticsPlayground/Utilities and Hardware/Latch ==
  note: Switch between 0 and 1 with every rising edge transition of the input trigger signal.
      |
      | The output toggles between 0 and 1 when the input is a rising signal (for example when a button is pressed). The output remains the same until the input rises again (for example, the button is pressed again).
  In : Inport
  Latch : Stateflow chart  TreatAsAtomicUnit=on
  Out : Outport
  wires:
  In/1 -> Latch/1(trigger)
  Latch/1(output) -> Out/1

== system RoboticsPlayground/Utilities and Hardware/More Controls (Double-Click) ==

== system RoboticsPlayground/Utilities and Hardware/Open//Get Support for Arduino (Double-click) ==

== system RoboticsPlayground/Utilities and Hardware/Open//Get Support for LEGO (Double-click) ==

== system RoboticsPlayground/Utilities and Hardware/Open//Get Support for VEX (Double-click) ==

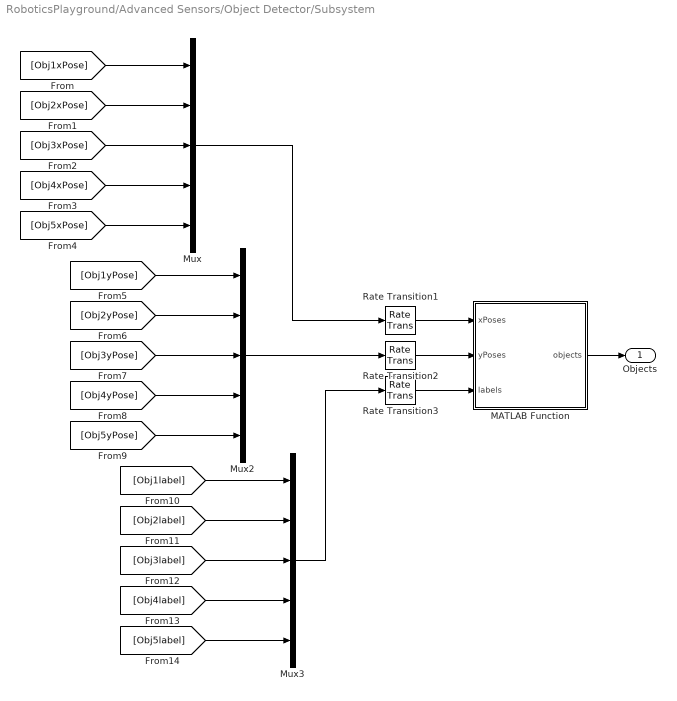
== system RoboticsPlayground/Advanced Sensors/Object Detector/Subsystem ==
  MATLAB Function : MATLAB Function  TreatAsAtomicUnit=on
  Mux : Mux  Inputs=5
  Mux2 : Mux  Inputs=5
  Mux3 : Mux  Inputs=5
  Rate Transition1 : RateTransition  OutPortSampleTime=sensorTs
  Rate Transition2 : RateTransition  OutPortSampleTime=sensorTs
  Rate Transition3 : RateTransition  OutPortSampleTime=sensorTs
  Objects : Outport  VectorParamsAs1DForOutWhenUnconnected=off
  wires:
  [Obj1xPose] -> Mux/1
  [Obj2xPose] -> Mux/2
  [Obj3xPose] -> Mux/3
  [Obj4xPose] -> Mux/4
  [Obj5xPose] -> Mux/5
  [Obj5yPose] -> Mux2/5
  [Obj4yPose] -> Mux2/4
  [Obj3yPose] -> Mux2/3
  [Obj2yPose] -> Mux2/2
  [Obj1yPose] -> Mux2/1
  [Obj1label] -> Mux3/1
  [Obj2label] -> Mux3/2
  [Obj3label] -> Mux3/3
  [Obj4label] -> Mux3/4
  [Obj5label] -> Mux3/5
  Mux2/1 -> Rate Transition2/1
  Mux/1 -> Rate Transition1/1
  Mux3/1 -> Rate Transition3/1
  MATLAB Function/1(objects) -> Objects/1
  Rate Transition1/1 -> MATLAB Function/1(xPoses)
  Rate Transition2/1 -> MATLAB Function/2(yPoses)
  Rate Transition3/1 -> MATLAB Function/3(labels)
